simulink library "vip"  (Simulink 8.1)
settings: Solver=ode45  StartTime=0.0  StopTime=10.0  RelTol=1e-3
undefined symbols (not defined in the file or in its folder): C_TASK_100MS_S, C_TICK_TIME_S, KAPP_SteeringRatio_rat, KAPP_WheelBase_m, KIFO_DefaultTurnRad_m, KIFO_HostVehicleWidth_m, KIFO_StraightSWARollAvg_deg, KIFO_StraightYawRate_degps, KIFO_TargInPathLatOffsetACC_m, KIFO_TargInPathLatOffsetAEB_m, KIFO_TargInPathLatOffsetFCW_m, TRUE, ZERO_FLOAT
libraries: hcu_lib x5, simulink x3, vil x1
settings Model: Creator=xsellart  LastModifiedBy=tescamilla

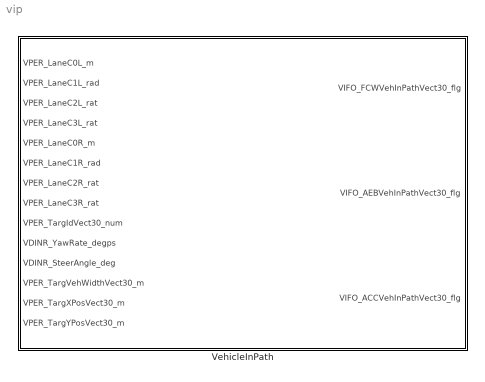
== system vip ==
  VehicleInPath : Subsystem

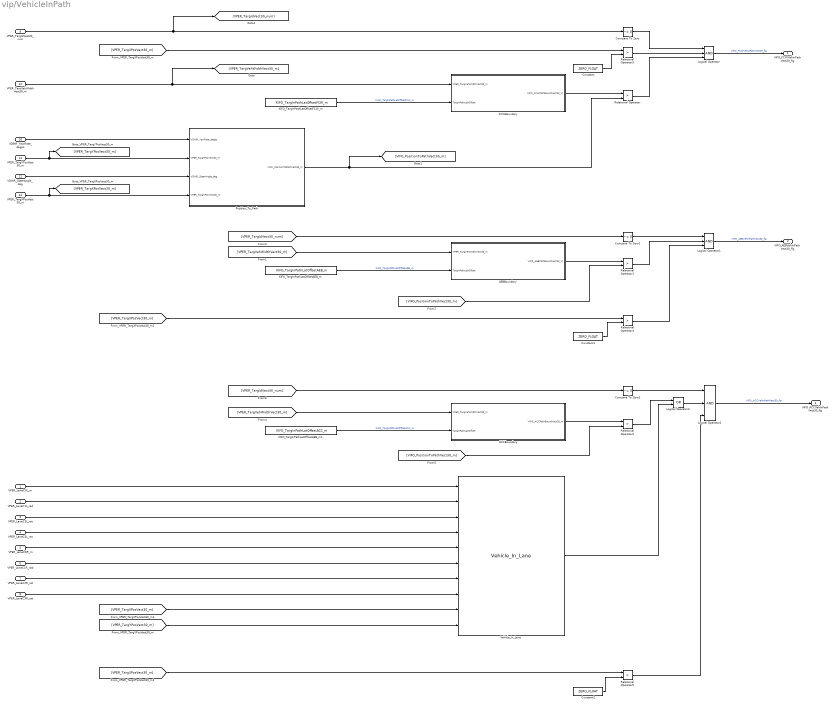
== system vip/VehicleInPath ==
  VPER_LaneC0L_m : Inport
  VPER_LaneC1L_rad : Inport  Port=2
  VPER_LaneC2L_rat : Inport  Port=3
  VPER_LaneC3L_rat : Inport  Port=4
  VPER_LaneC0R_m : Inport  Port=5
  VPER_LaneC1R_rad : Inport  Port=6
  VPER_LaneC2R_rat : Inport  Port=7
  VPER_LaneC3R_rat : Inport  Port=8
  VPER_TargIdVect30_num : Inport  Port=9
  VDINR_YawRate_degps : Inport  Port=10
  VDINR_SteerAngle_deg : Inport  Port=11
  VPER_TargVehWidthVect30_m : Inport  Port=12
  VPER_TargXPosVect30_m : Inport  Port=13
  VPER_TargYPosVect30_m : Inport  Port=14
  ACCBoundary : Subsystem
  AEBBoundary : Subsystem
  Compare To Zero : simulink/Logic and Bit Operations/Compare To Zero  relop=~=  OutDataTypeStr=boolean
  Compare To Zero1 : simulink/Logic and Bit Operations/Compare To Zero  relop=~=  OutDataTypeStr=boolean
  Compare To Zero2 : simulink/Logic and Bit Operations/Compare To Zero  relop=~=  OutDataTypeStr=boolean
  Constant : Constant  Value=ZERO_FLOAT
  Constant1 : Constant  Value=ZERO_FLOAT
  Constant2 : Constant  Value=ZERO_FLOAT
  FCWBoundary : Subsystem
  KIFO_TargInPathLatOffsetAEB_m : Constant  Value=KIFO_TargInPathLatOffsetAEB_m
  KIFO_TargInPathLatOffsetAEB_m1 : Constant  Value=KIFO_TargInPathLatOffsetACC_m
  KIFO_TargInPathLatOffsetFCW_m : Constant  Value=KIFO_TargInPathLatOffsetFCW_m
  Logical Operator : Logic  Inputs=3  AllPortsSameDT=off  OutDataTypeStr=boolean
  Logical Operator1 : Logic  Inputs=3  AllPortsSameDT=off  OutDataTypeStr=boolean
  Logical Operator2 : Logic  Inputs=3  AllPortsSameDT=off  OutDataTypeStr=boolean
  Logical Operator3 : Logic  Operator=OR  AllPortsSameDT=off  OutDataTypeStr=boolean
  Position_To_Path : Subsystem
  Relational Operator{,1..5} (6 alike) : RelationalOperator  Operator=>  OutDataTypeStr=boolean
  Vehicle_In_Lane : vil/Vehicle_In_Lane
  VIFO_FCWVehInPathVect30_flg : Outport
  VIFO_AEBVehInPathVect30_flg : Outport  Port=2
  VIFO_ACCVehInPathVect30_flg : Outport  Port=3
  wires:
  KIFO_TargInPathLatOffsetAEB_m1/1 -> ACCBoundary/2(TargInPathLatOffset)  "KIFO_TargInPathLatOffsetACC_m"
  [VIFO_PositionToPathVect30_m] -> Relational Operator2/2
  ACCBoundary/1(VIFO_ACCPathBoundVect30_m) -> Relational Operator2/1
  [VPER_TargVehWidthVect30_m] -> ACCBoundary/1(VPER_TargVehWidthVect30_m)
  [VPER_TargIdVect30_num] -> Compare To Zero2/1
  Compare To Zero2/1 -> Logical Operator2/1
  VPER_TargVehWidthVect30_m/1 -> [VPER_TargVehWidthVect30_m], FCWBoundary/1(VPER_TargVehWidthVect30_m)
  KIFO_TargInPathLatOffsetAEB_m/1 -> AEBBoundary/2(TargInPathLatOffset)  "KIFO_TargInPathLatOffsetAEB_m"
  VDINR_YawRate_degps/1 -> Position_To_Path/1(VDINR_YawRate_degps)
  [VIFO_PositionToPathVect30_m] -> Relational Operator1/2
  AEBBoundary/1(VIFO_AEBPathBoundVect30_m) -> Relational Operator1/1
  FCWBoundary/1(VIFO_FCWPathBoundVect30_m) -> Relational Operator/1
  [VPER_TargVehWidthVect30_m] -> AEBBoundary/1(VPER_TargVehWidthVect30_m)
  Position_To_Path/1(VIFO_PositionToPathVect30_m) -> Relational Operator/2, [VIFO_PositionToPathVect30_m]
  KIFO_TargInPathLatOffsetFCW_m/1 -> FCWBoundary/2(TargInPathLatOffset)  "KIFO_TargInPathLatOffsetFCW_m"
  VPER_TargYPosVect30_m/1 -> Position_To_Path/2(VPER_TargYPosVect30_m), [VPER_TargYPosVect30_m]
  VDINR_SteerAngle_deg/1 -> Position_To_Path/3(VDINR_SteerAngle_deg)
  VPER_TargXPosVect30_m/1 -> Position_To_Path/4(VPER_TargXPosVect30_m), [VPER_TargXPosVect30_m]
  VPER_TargIdVect30_num/1 -> [VPER_TargIdVect30_num], Compare To Zero/1
  Compare To Zero/1 -> Logical Operator/1
  Logical Operator/1 -> VIFO_FCWVehInPathVect30_flg/1  "VIFO_FCWVehInPathVect30_flg"
  Relational Operator/1 -> Logical Operator/3
  [VPER_TargIdVect30_num] -> Compare To Zero1/1
  Logical Operator1/1 -> VIFO_AEBVehInPathVect30_flg/1  "VIFO_AEBVehInPathVect30_flg"
  Compare To Zero1/1 -> Logical Operator1/1
  Relational Operator1/1 -> Logical Operator1/2
  [VPER_TargXPosVect30_m] -> Relational Operator3/1
  Constant/1 -> Relational Operator3/2
  Relational Operator3/1 -> Logical Operator/2
  [VPER_TargXPosVect30_m] -> Relational Operator4/1
  Constant1/1 -> Relational Operator4/2
  [VPER_TargXPosVect30_m] -> Relational Operator5/1
  Constant2/1 -> Relational Operator5/2
  Relational Operator4/1 -> Logical Operator1/3
  Relational Operator5/1 -> Logical Operator2/3
  Vehicle_In_Lane/1 -> Logical Operator3/2
  [VPER_TargXPosVect30_m] -> Vehicle_In_Lane/9
  [VPER_TargYPosVect30_m] -> Vehicle_In_Lane/10
  VPER_LaneC0L_m/1 -> Vehicle_In_Lane/1
  VPER_LaneC1R_rad/1 -> Vehicle_In_Lane/6
  VPER_LaneC3L_rat/1 -> Vehicle_In_Lane/4
  VPER_LaneC2L_rat/1 -> Vehicle_In_Lane/3
  VPER_LaneC1L_rad/1 -> Vehicle_In_Lane/2
  VPER_LaneC0R_m/1 -> Vehicle_In_Lane/5
  VPER_LaneC3R_rat/1 -> Vehicle_In_Lane/8
  VPER_LaneC2R_rat/1 -> Vehicle_In_Lane/7
  Logical Operator2/1 -> VIFO_ACCVehInPathVect30_flg/1  "VIFO_ACCVehInPathVect30_flg"
  Relational Operator2/1 -> Logical Operator3/1
  Logical Operator3/1 -> Logical Operator2/2

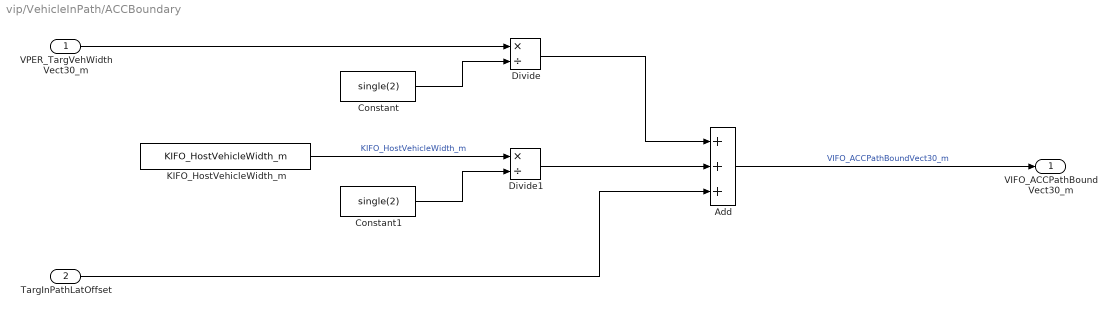
== system vip/VehicleInPath/ACCBoundary ==
  VPER_TargVehWidthVect30_m : Inport
  TargInPathLatOffset : Inport  Port=2
  Add : Sum  Inputs=+++
  Constant : Constant  Value=single(2)  OutDataTypeStr=single
  Constant1 : Constant  Value=single(2)  OutDataTypeStr=single
  Divide : Product  Inputs=*/
  Divide1 : Product  Inputs=*/
  KIFO_HostVehicleWidth_m : Constant  Value=KIFO_HostVehicleWidth_m
  VIFO_ACCPathBoundVect30_m : Outport
  wires:
  VPER_TargVehWidthVect30_m/1 -> Divide/1
  Divide/1 -> Add/1
  Constant1/1 -> Divide1/2
  Divide1/1 -> Add/2
  Add/1 -> VIFO_ACCPathBoundVect30_m/1  "VIFO_ACCPathBoundVect30_m"
  KIFO_HostVehicleWidth_m/1 -> Divide1/1  "KIFO_HostVehicleWidth_m"
  TargInPathLatOffset/1 -> Add/3
  Constant/1 -> Divide/2

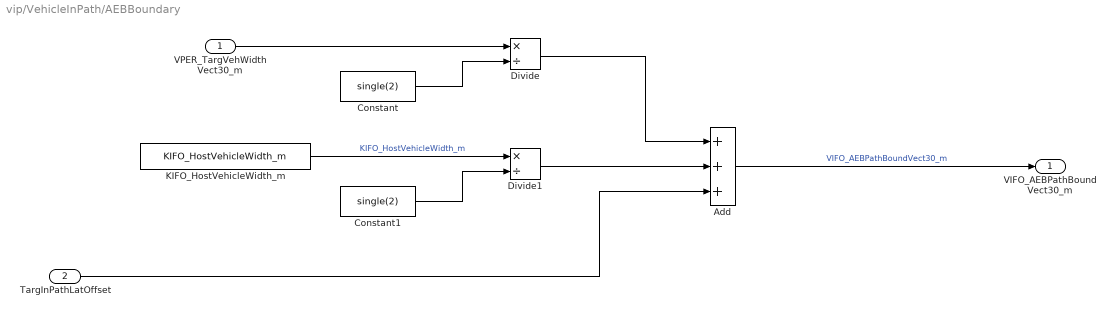
== system vip/VehicleInPath/AEBBoundary ==
  VPER_TargVehWidthVect30_m : Inport
  TargInPathLatOffset : Inport  Port=2
  Add : Sum  Inputs=+++
  Constant : Constant  Value=single(2)  OutDataTypeStr=single
  Constant1 : Constant  Value=single(2)  OutDataTypeStr=single
  Divide : Product  Inputs=*/
  Divide1 : Product  Inputs=*/
  KIFO_HostVehicleWidth_m : Constant  Value=KIFO_HostVehicleWidth_m
  VIFO_AEBPathBoundVect30_m : Outport
  wires:
  VPER_TargVehWidthVect30_m/1 -> Divide/1
  Divide/1 -> Add/1
  Constant1/1 -> Divide1/2
  Divide1/1 -> Add/2
  Add/1 -> VIFO_AEBPathBoundVect30_m/1  "VIFO_AEBPathBoundVect30_m"
  KIFO_HostVehicleWidth_m/1 -> Divide1/1  "KIFO_HostVehicleWidth_m"
  TargInPathLatOffset/1 -> Add/3
  Constant/1 -> Divide/2

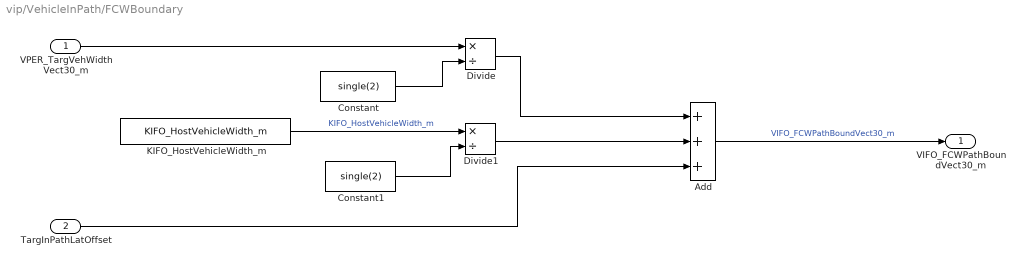
== system vip/VehicleInPath/FCWBoundary ==
  VPER_TargVehWidthVect30_m : Inport
  TargInPathLatOffset : Inport  Port=2
  Add : Sum  Inputs=+++
  Constant : Constant  Value=single(2)  OutDataTypeStr=single
  Constant1 : Constant  Value=single(2)  OutDataTypeStr=single
  Divide : Product  Inputs=*/
  Divide1 : Product  Inputs=*/
  KIFO_HostVehicleWidth_m : Constant  Value=KIFO_HostVehicleWidth_m
  VIFO_FCWPathBoundVect30_m : Outport
  wires:
  Constant/1 -> Divide/2
  TargInPathLatOffset/1 -> Add/3
  KIFO_HostVehicleWidth_m/1 -> Divide1/1  "KIFO_HostVehicleWidth_m"
  Add/1 -> VIFO_FCWPathBoundVect30_m/1  "VIFO_FCWPathBoundVect30_m"
  Divide1/1 -> Add/2
  Constant1/1 -> Divide1/2
  Divide/1 -> Add/1
  VPER_TargVehWidthVect30_m/1 -> Divide/1

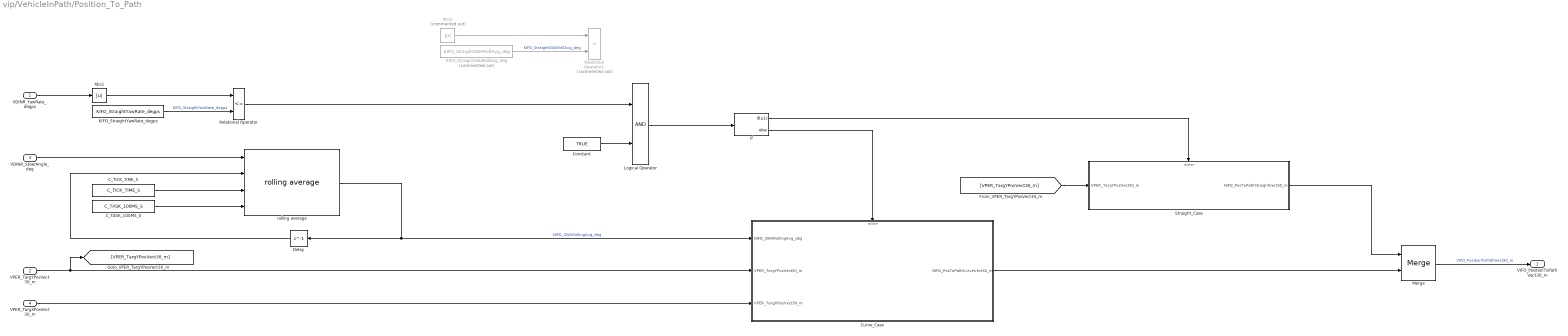
== system vip/VehicleInPath/Position_To_Path ==
  VDINR_YawRate_degps : Inport
  VPER_TargYPosVect30_m : Inport  Port=2  PortDimensions=30
  VDINR_SteerAngle_deg : Inport  Port=3
  VPER_TargXPosVect30_m : Inport  Port=4  PortDimensions=30
  Abs1 : Abs
  Abs2 : Abs  Commented=on
  C_TASK_100MS_S : Constant  Value=C_TASK_100MS_S
  C_TICK_TIME_S : Constant  Value=C_TICK_TIME_S
  Constant : Constant  Value=TRUE
  Curve_Case : Subsystem  TreatAsAtomicUnit=on
  Delay : Delay  DelayLength=1
  If : If  IfExpression=u1
  KIFO_StraightSWARollAvg_deg : Constant  Commented=on  Value=KIFO_StraightSWARollAvg_deg
  KIFO_StraightYawRate_degps : Constant  Value=KIFO_StraightYawRate_degps
  Logical Operator : Logic  AllPortsSameDT=off  OutDataTypeStr=boolean
  Merge : Merge
  Relational Operator : RelationalOperator  Operator=<=  OutDataTypeStr=boolean
  Relational Operator1 : RelationalOperator  Commented=on  Operator=<  OutDataTypeStr=boolean
  Straight_Case : Subsystem  TreatAsAtomicUnit=on
  rolling average : hcu_lib/rolling average
  VIFO_PositionToPathVect30_m : Outport
  wires:
  Curve_Case/1(NIFO_PosToPathCurveVect30_m) -> Merge/2
  Merge/1 -> VIFO_PositionToPathVect30_m/1  "VIFO_PositionToPathVect30_m"
  VPER_TargYPosVect30_m/1 -> [VPER_TargYPosVect30_m], Curve_Case/2(VPER_TargYPosVect30_m)
  Straight_Case/1(NIFO_PosToPathStraightVect30_m) -> Merge/1
  VPER_TargXPosVect30_m/1 -> Curve_Case/3(VPER_TargXPosVect30_m)
  If/1 -> Straight_Case/Action
  [VPER_TargYPosVect30_m] -> Straight_Case/1(VPER_TargYPosVect30_m)
  If/2 -> Curve_Case/Action
  VDINR_YawRate_degps/1 -> Abs1/1
  Abs1/1 -> Relational Operator/1
  KIFO_StraightYawRate_degps/1 -> Relational Operator/2  "KIFO_StraightYawRate_degps"
  VDINR_SteerAngle_deg/1 -> rolling average/1
  C_TICK_TIME_S/1 -> rolling average/3
  C_TASK_100MS_S/1 -> rolling average/4
  rolling average/1 -> Curve_Case/1(NIFO_SWARollingAvg_deg), Delay/1  "NIFO_SWARollingAvg_deg"
  KIFO_StraightSWARollAvg_deg/1 -> Relational Operator1/2  "KIFO_StraightSWARollAvg_deg"
  Relational Operator/1 -> Logical Operator/1
  Logical Operator/1 -> If/1
  Abs2/1 -> Relational Operator1/1
  Delay/1 -> rolling average/2
  Constant/1 -> Logical Operator/2

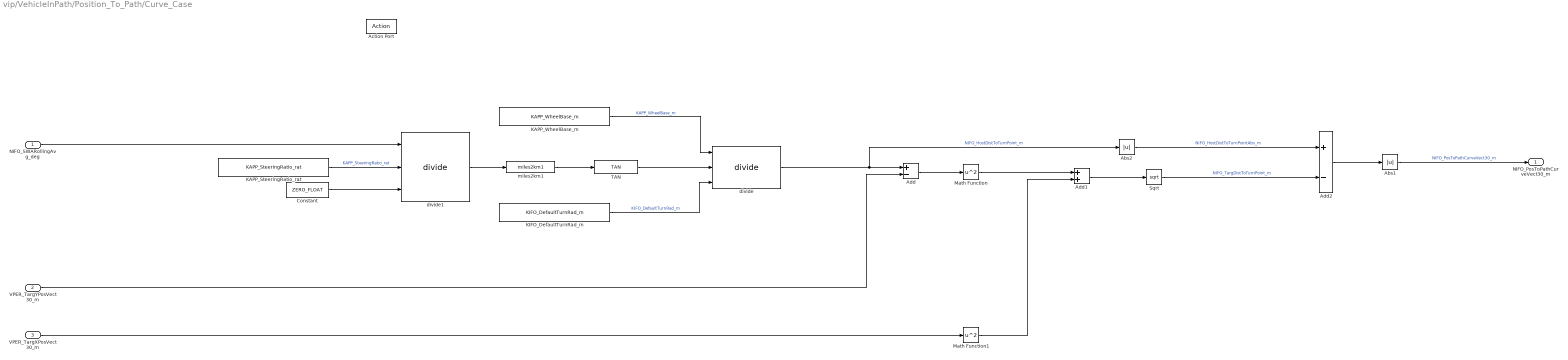
== system vip/VehicleInPath/Position_To_Path/Curve_Case ==
  NIFO_SWARollingAvg_deg : Inport
  VPER_TargYPosVect30_m : Inport  Port=2
  VPER_TargXPosVect30_m : Inport  Port=3
  Action Port : ActionPort
  Abs1 : Abs
  Abs2 : Abs
  Add : Sum  Inputs=+-
  Add1 : Sum
  Add2 : Sum  Inputs=+-
  Constant : Constant  Value=ZERO_FLOAT
  KAPP_SteeringRatio_rat : Constant  Value=KAPP_SteeringRatio_rat
  KAPP_WheelBase_m : Constant  Value=KAPP_WheelBase_m
  KIFO_DefaultTurnRad_m : Constant  Value=KIFO_DefaultTurnRad_m
  Math Function : Math  Operator=square  SaturateOnIntegerOverflow=on
  Math Function1 : Math  Operator=square  SaturateOnIntegerOverflow=on
  Sqrt : Sqrt  SaturateOnIntegerOverflow=on
  TAN : hcu_lib/TAN
  divide : hcu_lib/divide
  divide1 : hcu_lib/divide
  miles2km1 : hcu_lib/miles2km1
  NIFO_PosToPathCurveVect30_m : Outport
  wires:
  Abs2/1 -> Add2/1  "NIFO_HostDistToTurnPointAbs_m"
  KAPP_WheelBase_m/1 -> divide/1  "KAPP_WheelBase_m"
  KAPP_SteeringRatio_rat/1 -> divide1/2  "KAPP_SteeringRatio_rat"
  KIFO_DefaultTurnRad_m/1 -> divide/3  "KIFO_DefaultTurnRad_m"
  VPER_TargYPosVect30_m/1 -> Add/2
  divide/1 -> Add/1, Abs2/1  "NIFO_HostDistToTurnPoint_m"
  Add/1 -> Math Function/1
  VPER_TargXPosVect30_m/1 -> Math Function1/1
  Math Function/1 -> Add1/1
  Math Function1/1 -> Add1/2
  Add1/1 -> Sqrt/1
  Sqrt/1 -> Add2/2  "NIFO_TargDistToTurnPoint_m"
  Add2/1 -> Abs1/1
  Abs1/1 -> NIFO_PosToPathCurveVect30_m/1  "NIFO_PosToPathCurveVect30_m"
  TAN/1 -> divide/2
  miles2km1/1 -> TAN/1
  divide1/1 -> miles2km1/1
  Constant/1 -> divide1/3
  NIFO_SWARollingAvg_deg/1 -> divide1/1

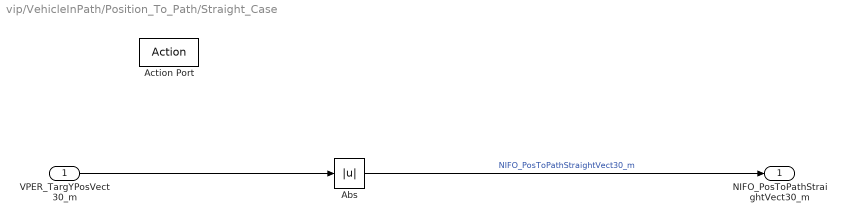
== system vip/VehicleInPath/Position_To_Path/Straight_Case ==
  VPER_TargYPosVect30_m : Inport
  Action Port : ActionPort
  Abs : Abs
  NIFO_PosToPathStraightVect30_m : Outport
  wires:
  Abs/1 -> NIFO_PosToPathStraightVect30_m/1  "NIFO_PosToPathStraightVect30_m"
  VPER_TargYPosVect30_m/1 -> Abs/1
